simulink model "untitled"  (R2020a)
settings: Solver=VariableStepAuto  StartTime=0.0  StopTime=10.0  RelTol=1e-3
values from neighbouring files (symbols this model uses):
  k1 = 1.6e4    (= 16000)    [Problema1.m]    (also in Problema2A.m = 3)
  k2 = 1.6e5    (= 160000)    [Problema1.m]    (also in Problema2A.m = 1.5)
  k3 = 2.3    [Problema2A.m]
  k4 = 1.8    [Problema2A.m]
settings Model: OrderedModelArguments=off  Creator=Usuario  LastModifiedBy=Usuario

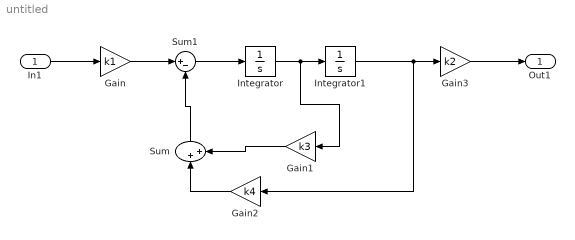
== system untitled ==
  In1 : Inport
  Gain : Gain  Gain=k1
  Gain1 : Gain  Gain=k3
  Gain2 : Gain  Gain=k4
  Gain3 : Gain  Gain=k2
  Integrator : Integrator
  Integrator1 : Integrator
  Sum : Sum  Inputs=|++
  Sum1 : Sum  Inputs=|+-
  Out1 : Outport
  wires:
  Integrator/1 -> Gain1/1, Integrator1/1
  Integrator1/1 -> Gain3/1, Gain2/1
  Sum/1 -> Sum1/2
  Sum1/1 -> Integrator/1
  Gain/1 -> Sum1/1
  In1/1 -> Gain/1
  Gain3/1 -> Out1/1
  Gain1/1 -> Sum/2
  Gain2/1 -> Sum/1
